simulink model "simCG"  (R2015a)
settings: Solver=ode4  SolverMode=SingleTasking  StartTime=0.0  StopTime=10.0  FixedStep=0.01  RelTol=1e-3
values from neighbouring files (symbols this model uses):
  A_Wd = T*((Hc*invPhi*G) + L)    [CG_Offline.m]
  AW_Vx = [AW_Vx; T*(Rkc{t})]    [CG_Offline.m]
  Ax_Vx = [Ax_Vx; T*Hc*(Phi^t)]    [CG_Offline.m]
  b_Vx = repmat(b, (k0+1),1)    [CG_Offline.m]
  b_Wd = b - delta*sqrt(proj)    [CG_Offline.m]
  dda_max = 2.50    (= 2.5)    [Main.m]    (also in main_CG.m)
  Kd_fb = Kd(:,1:nx)    [Main.m]    (also in main_CG.m; main_TD.m)
  nx = size(Phi,1)    [CG_Offline.m]
  Psi = eye(ng)    [Main.m]    (also in main_CG.m)
  Ts = 0.01    [Main.m]    (also in main_CG.m; main_TC.m; main_TD.m)
undefined symbols (not defined in the file or in its folder): Ad, Adi, Bd, Bdi, Cdi, CG, Ddi, nu
settings Model: CovSFcnEnable=off  Creator=pier  LastModifiedBy=Piero
settings OptimizationCC: BlockReduction=off  BooleanDataType=off
settings DebuggingCC: SaveWithParameterizedLinksMsg=none  UnderspecifiedInitializationDetection=Classic  MergeDetectMultiDrivingBlocksExec=none  SignalResolutionControl=TryResolveAllWithWarning
settings HardwareCC: TargetUnknown=on

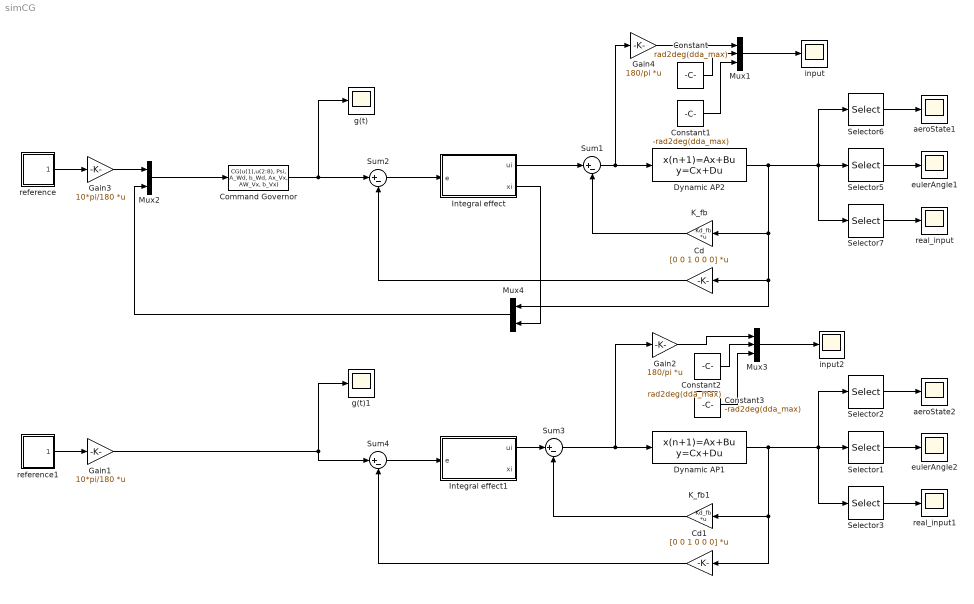
== system simCG ==
  Cd : Gain  Gain=[0 0 1 0 0 0]  Multiplication=Matrix(K*u)
  Cd1 : Gain  Gain=[0 0 1 0 0 0]  Multiplication=Matrix(K*u)
  Command Governor : MATLABFcn  MATLABFcn=CG(u(1),u(2:8), Psi, A_Wd, b_Wd, Ax_Vx, AW_Vx, b_Vx)  OutputDimensions=1
  Constant : Constant  Value=rad2deg(dda_max)
  Constant1 : Constant  Value=-rad2deg(dda_max)
  Constant2 : Constant  Value=rad2deg(dda_max)
  Constant3 : Constant  Value=-rad2deg(dda_max)
  Dynamic AP1 : DiscreteStateSpace  A=Ad  B=Bd  C=eye(nx)  D=zeros(nx,nu)  SampleTime=Ts
  Dynamic AP2 : DiscreteStateSpace  A=Ad  B=Bd  C=eye(nx)  D=zeros(nx,nu)  SampleTime=Ts
  Gain1 : Gain  Gain=10*pi/180  Multiplication=Matrix(K*u)
  Gain2 : Gain  Gain=180/pi  Multiplication=Matrix(K*u)
  Gain3 : Gain  Gain=10*pi/180  Multiplication=Matrix(K*u)
  Gain4 : Gain  Gain=180/pi  Multiplication=Matrix(K*u)
  Integral effect : Subsystem
  Integral effect1 : Subsystem
  K_fb : Gain  Gain=Kd_fb  Multiplication=Matrix(K*u)
  K_fb1 : Gain  Gain=Kd_fb  Multiplication=Matrix(K*u)
  Mux1 : Mux  Inputs=3
  Mux2 : Mux  Inputs=2
  Mux3 : Mux  Inputs=3
  Mux4 : Mux  Inputs=2
  Selector1 : Selector  InputPortWidth=6  Indices=[3:4]
  Selector2 : Selector  InputPortWidth=6  Indices=[1:2]
  Selector3 : Selector  InputPortWidth=6  Indices=[5:6]
  Selector5 : Selector  InputPortWidth=6  Indices=[3:4]
  Selector6 : Selector  InputPortWidth=6  Indices=[1:2]
  Selector7 : Selector  InputPortWidth=6  Indices=[5:6]
  Sum{1..4} (4 alike) : Sum  Inputs=|+-
  aeroState1 : Scope
      settings: TimeRange=100  SaveName=sim_aeroState
  aeroState2 : Scope
      settings: TimeRange=100  SaveName=sim_aeroState1
  eulerAngle1 : Scope
      settings: TimeRange=10  YMin=-0.025  YMax=0.275  SaveName=sim_eulerAngles
  eulerAngle2 : Scope
      settings: TimeRange=10  YMin=-0.025  YMax=0.275  SaveName=sim_eulerAngles1
  g(t) : Scope
      settings: YMin=0.0829032  YMax=0.0916298
  g(t)1 : Scope
      settings: YMin=0.0829032  YMax=0.0916298
  input : Scope
      settings: YMin=-0.55  YMax=0.45  SampleInput=on  SampleTime=0.01
  input2 : Scope
      settings: YMin=-0.55  YMax=0.45  SaveName=ScopeData3  SampleInput=on  SampleTime=0.01
  real_input : Scope
      settings: SaveName=sim_realInput  SampleInput=on  SampleTime=Ts
  real_input1 : Scope
      settings: SaveName=sim_realInput1  SampleInput=on  SampleTime=Ts
  reference : Subsystem
  reference1 : Subsystem
  wires:
  Sum1/1 -> Dynamic AP2/1, Gain4/1
  K_fb/1 -> Sum1/2
  Cd/1 -> Sum2/2
  Sum2/1 -> Integral effect/1(e)
  Integral effect/1(ui) -> Sum1/1
  Integral effect/2(xi) -> Mux4/2
  Mux2/1 -> Command Governor/1
  Command Governor/1 -> g(t)/1, Sum2/1
  Mux4/1 -> Mux2/2
  reference/1(Out1) -> Gain3/1
  Gain3/1 -> Mux2/1
  Selector5/1 -> eulerAngle1/1
  Selector7/1 -> real_input/1
  Selector6/1 -> aeroState1/1
  Dynamic AP2/1 -> Selector7/1, Selector5/1, Selector6/1, K_fb/1, Cd/1, Mux4/1
  Sum3/1 -> Gain2/1, Dynamic AP1/1
  K_fb1/1 -> Sum3/2
  Cd1/1 -> Sum4/2
  Sum4/1 -> Integral effect1/1(e)
  Integral effect1/1(ui) -> Sum3/1
  Gain1/1 -> Sum4/1, g(t)1/1
  reference1/1(Out1) -> Gain1/1
  Selector1/1 -> eulerAngle2/1
  Selector3/1 -> real_input1/1
  Selector2/1 -> aeroState2/1
  Dynamic AP1/1 -> Cd1/1, K_fb1/1, Selector2/1, Selector1/1, Selector3/1
  Gain4/1 -> Mux1/1
  Mux1/1 -> input/1
  Constant/1 -> Mux1/2
  Constant1/1 -> Mux1/3
  Gain2/1 -> Mux3/1
  Mux3/1 -> input2/1
  Constant2/1 -> Mux3/2
  Constant3/1 -> Mux3/3

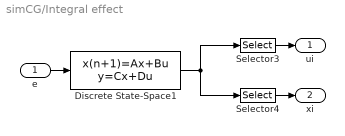
== system simCG/Integral effect ==
  e : Inport
  Discrete State-Space1 : DiscreteStateSpace  A=Adi  B=Bdi  C=[Cdi; 1]  D=[Ddi; 0]  SampleTime=Ts
  Selector3 : Selector  InputPortWidth=3  Indices=[1 2]
  Selector4 : Selector  InputPortWidth=3  Indices=[3]
  ui : Outport
  xi : Outport  Port=2
  wires:
  e/1 -> Discrete State-Space1/1
  Selector4/1 -> xi/1
  Selector3/1 -> ui/1
  Discrete State-Space1/1 -> Selector3/1, Selector4/1

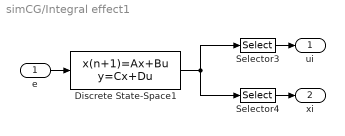
== system simCG/Integral effect1 ==
  e : Inport
  Discrete State-Space1 : DiscreteStateSpace  A=Adi  B=Bdi  C=[Cdi; 1]  D=[Ddi; 0]  SampleTime=Ts
  Selector3 : Selector  InputPortWidth=3  Indices=[1 2]
  Selector4 : Selector  InputPortWidth=3  Indices=[3]
  ui : Outport
  xi : Outport  Port=2
  wires:
  Discrete State-Space1/1 -> Selector4/1, Selector3/1
  Selector3/1 -> ui/1
  Selector4/1 -> xi/1
  e/1 -> Discrete State-Space1/1

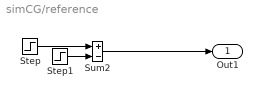
== system simCG/reference ==
  Step : Step  Time=2.5  SampleTime=0
  Step1 : Step  Time=12.5  SampleTime=0
  Sum2 : Sum  Inputs=+-
  Out1 : Outport
  wires:
  Sum2/1 -> Out1/1
  Step/1 -> Sum2/1
  Step1/1 -> Sum2/2

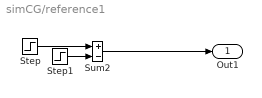
== system simCG/reference1 ==
  Step : Step  Time=2.5  SampleTime=0
  Step1 : Step  Time=12.5  SampleTime=0
  Sum2 : Sum  Inputs=+-
  Out1 : Outport
  wires:
  Step1/1 -> Sum2/2
  Step/1 -> Sum2/1
  Sum2/1 -> Out1/1
